simulink library "discreteSecondOrderPD_cl"  (R2022a)
settings: Solver=VariableStepAuto  StartTime=0.0  StopTime=10.0  RelTol=1e-3
undefined symbols (not defined in the file): Ts
libraries: discreteFilter_ul x1
settings Model: Creator=adabney  LastModifiedBy=adabney

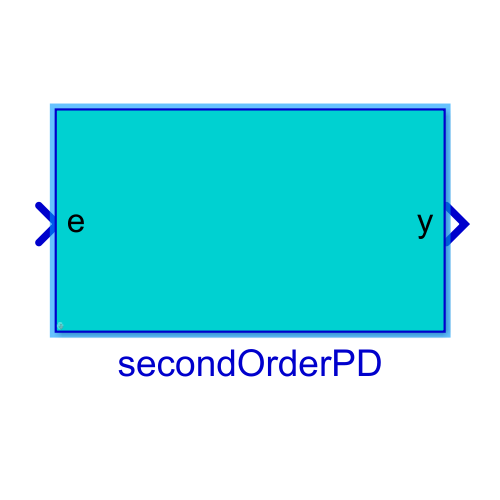
[thumbnail: Simulink's stored preview of the top-level diagram]
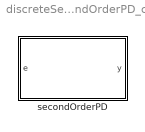
== system discreteSecondOrderPD_cl ==
  secondOrderPD : Subsystem  mask{kP=0, kD=0, tauReference=0, tauDerivative=1, Ts=Ts}
      mask prompts: kP "Proportional Gain"; kD "Derivative Gain"; tauReference "Reference Filter Time Constant"; tauDerivative "Derivative Filter Time Constant"; Ts "Sample Time"
      mask DialogControl DescTextVar Prompt: Mask for inputting controller gains for a second order filtered PD controller
      mask DialogControl ParameterGroupVar Prompt: Gains

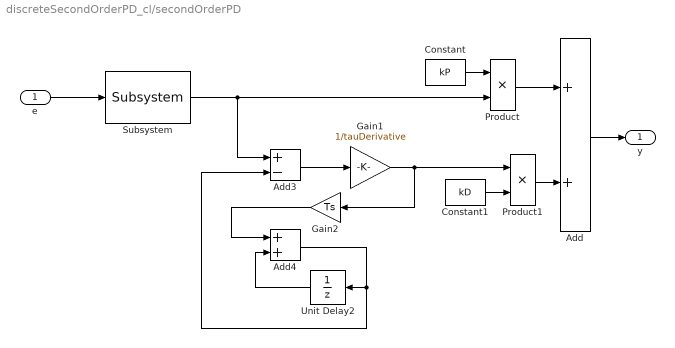
== system discreteSecondOrderPD_cl/secondOrderPD ==
  e : Inport
  Add : Sum
  Add3 : Sum  Inputs=+-
  Add4 : Sum
  Constant : Constant  Value=kP
  Constant1 : Constant  Value=kD
  Gain1 : Gain  Gain=1/tauDerivative
  Gain2 : Gain  Gain=Ts
  Product : Product
  Product1 : Product
  Subsystem : discreteFilter_ul/Subsystem  Ts=Ts  tau=tauReference
  Unit Delay2 : UnitDelay  SampleTime=-1  HasFrameUpgradeWarning=on
  y : Outport
  wires:
  e/1 -> Subsystem/1
  Gain1/1 -> Gain2/1, Product1/1
  Add/1 -> y/1
  Product/1 -> Add/1
  Product1/1 -> Add/2
  Constant1/1 -> Product1/2
  Constant/1 -> Product/1
  Gain2/1 -> Add4/1
  Add4/1 -> Add3/2, Unit Delay2/1
  Subsystem/1 -> Product/2, Add3/1
  Unit Delay2/1 -> Add4/2
  Add3/1 -> Gain1/1
